simulink model "BoostConverterMdl"  (R2015a)
settings: Solver=ode3  StartTime=0.0  StopTime=30  FixedStep=0.001  RelTol=1e-3
libraries: powerlib_meascontrol x1
settings Model: SimulationMode=accelerator  Creator=jreimers  LastModifiedBy=jreimers
settings DataIOCC: LimitDataPoints=off
settings HardwareCC: ProdBitPerChar=16  ProdBitPerInt=16  ProdBitPerPointer=16  ProdLargestAtomicInteger=Integer  ProdIntDivRoundTo=Zero  ProdEndianess=LittleEndian  ProdWordSize=16  ProdHWDeviceType=Texas Instruments->C2000

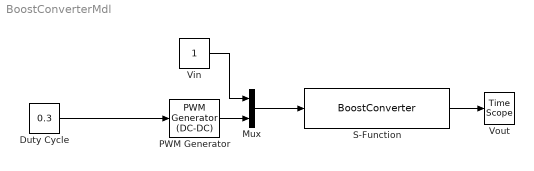
== system BoostConverterMdl ==
  Duty Cycle : Constant  Value=0.3
  Mux : Mux  Inputs=2
  PWM Generator : powerlib_meascontrol/Pulse & Signal Generators/PWM Generator (DC-DC)  Fsw=100  Ts=0
  S-Function : S-Function  FunctionName=BoostConverter
  Vin : Constant
  Vout : TimeScope
  wires:
  Vin/1 -> Mux/1
  Mux/1 -> S-Function/1
  Duty Cycle/1 -> PWM Generator/1
  PWM Generator/1 -> Mux/2
  S-Function/1 -> Vout/1
